simulink subsystem "fuel_ox_exhaustion"  (R2026a)
settings: Solver=VariableStepAuto
settings Model: Creator=ripro  LastModifiedBy=ripro

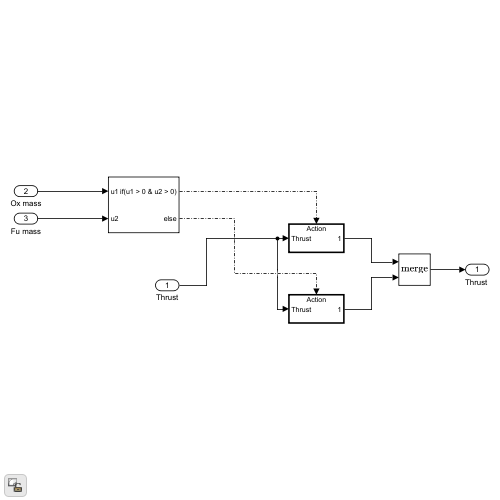
[thumbnail: Simulink's stored preview of the top-level diagram]
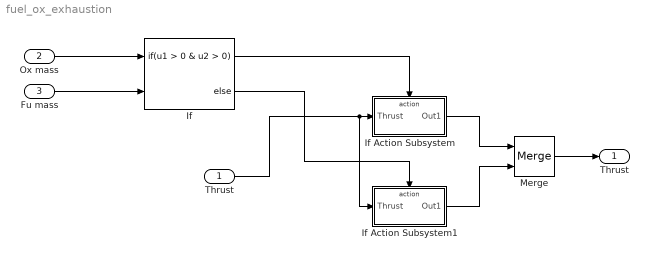
== system fuel_ox_exhaustion ==
  Thrust : Inport
  Ox mass : Inport  Port=2
  Fu mass : Inport  Port=3
  If : If  NumInputs=2  IfExpression=u1 > 0 & u2 > 0
  If Action Subsystem : Subsystem  TreatAsAtomicUnit=on
  If Action Subsystem1 : Subsystem  TreatAsAtomicUnit=on
  Merge : Merge
  "Thrust " : Outport
  wires:
  Ox mass/1 -> If/1
  Fu mass/1 -> If/2
  If/1 -> If Action Subsystem/Action
  If/2 -> If Action Subsystem1/Action
  Thrust/1 -> If Action Subsystem/1(Thrust), If Action Subsystem1/1(Thrust)
  If Action Subsystem/1(Out1) -> Merge/1
  If Action Subsystem1/1(Out1) -> Merge/2
  Merge/1 -> "Thrust "/1

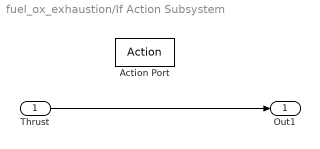
== system fuel_ox_exhaustion/If Action Subsystem ==
  Thrust : Inport
  Action Port : ActionPort
  Out1 : Outport
  wires:
  Thrust/1 -> Out1/1

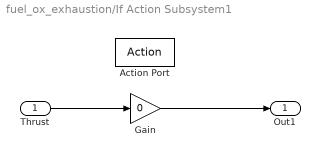
== system fuel_ox_exhaustion/If Action Subsystem1 ==
  Thrust : Inport
  Action Port : ActionPort
  Gain : Gain  Gain=0
  Out1 : Outport
  wires:
  Gain/1 -> Out1/1
  Thrust/1 -> Gain/1
